simulink model "SMC_4WS_JSY"  (R2020a)
settings: Solver=VariableStepAuto  StartTime=0.0  StopTime=10  RelTol=1e-3
values from neighbouring files (symbols this model uses):
  g = 9.8    [shuju.m]
  k = m/L*(-b/Kf+a/Kr)    (= 0.0025566955381)    [shuju.m]
  L = 2.91    [shuju.m]
  v = 108/3.6    (= 30)    [shuju.m]
libraries: Solver_SF x1
settings Model: Creator=wsj  LastModifiedBy=wsj

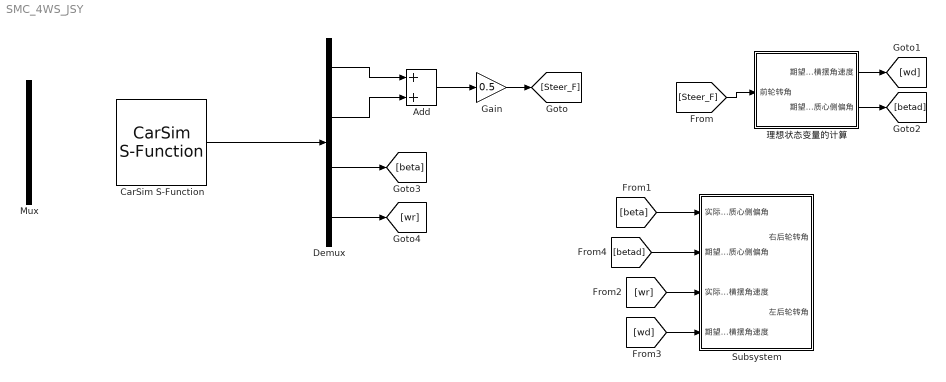
== system SMC_4WS_JSY ==
  Add : Sum
  CarSim S-Function : Solver_SF/CarSim S-Function  Priority=1  SIMFILE=simfile.sim  Run_RTs=off  vs_state_ind=Run  StopMode_ind=Vehicle Model
  Demux : Demux
  Gain : Gain  Gain=0.5
  Mux : Mux  Inputs=2
  Subsystem : Subsystem
  理想状态变量的计算 : Subsystem
  wires:
  Demux/1 -> Add/1
  Demux/2 -> Add/2
  Add/1 -> Gain/1
  CarSim S-Function/1 -> Demux/1
  Gain/1 -> [Steer_F]
  [Steer_F] -> 理想状态变量的计算/1(前轮转角)
  理想状态变量的计算/1(期望横摆角速度) -> [wd]
  理想状态变量的计算/2(期望质心侧偏角) -> [betad]
  Demux/4 -> [wr]
  Demux/3 -> [beta]
  [beta] -> Subsystem/1(实际质心侧偏角)
  [wr] -> Subsystem/3(实际横摆角速度)
  [wd] -> Subsystem/4(期望横摆角速度)
  [betad] -> Subsystem/2(期望质心侧偏角)

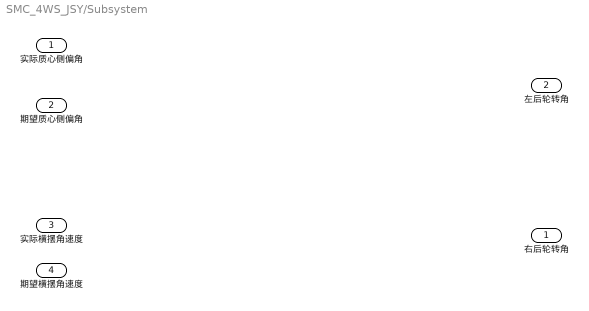
== system SMC_4WS_JSY/Subsystem ==
  实际质心侧偏角 : Inport
  期望质心侧偏角 : Inport  Port=2
  实际横摆角速度 : Inport  Port=3
  期望横摆角速度 : Inport  Port=4
  右后轮转角 : Outport
  左后轮转角 : Outport  Port=2

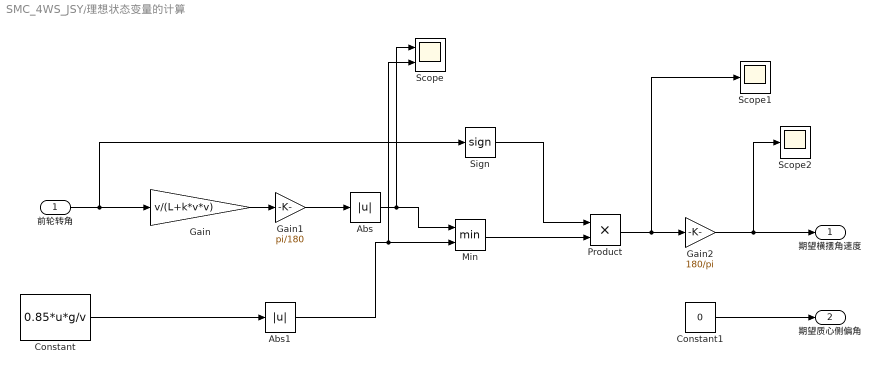
== system SMC_4WS_JSY/理想状态变量的计算 ==
  前轮转角 : Inport
  Abs : Abs
  Abs1 : Abs
  Constant : Constant  Value=0.85*u*g/v
  Constant1 : Constant  Value=0
  Gain : Gain  Gain=v/(L+k*v*v)
  Gain1 : Gain  Gain=pi/180
  Gain2 : Gain  Gain=180/pi
  Min : MinMax  Inputs=2
  Product : Product
  Scope : Scope  NumInputPorts=2
  Scope1 : Scope
  Scope2 : Scope
  Sign : Signum
  期望横摆角速度 : Outport
  期望质心侧偏角 : Outport  Port=2
  wires:
  前轮转角/1 -> Sign/1, Gain/1
  Gain/1 -> Gain1/1
  Gain1/1 -> Abs/1
  Abs/1 -> Scope/1, Min/1
  Constant/1 -> Abs1/1
  Abs1/1 -> Min/2, Scope/2
  Sign/1 -> Product/1
  Min/1 -> Product/2
  Product/1 -> Scope1/1, Gain2/1
  Gain2/1 -> Scope2/1, 期望横摆角速度/1
  Constant1/1 -> 期望质心侧偏角/1
